simulink model "rtwdemo_basicsc"  (Simulink 7.6)
settings: Solver=FixedStepDiscrete  StartTime=0.0  StopTime=10.0  FixedStep=1  RelTol=1e-3
PostLoadFcn:
  | open_system('rtwdemo_basicsc/Auto');
values from neighbouring files (symbols this model uses):
  K1 = 3    [rtwdemo_cgv_init.m]    (also in rtwdemo_dow_data.m)
undefined symbols (not defined in the file or in its folder): LOWER, T1Break, T1Data, T2Data, UPPER
libraries: rtwdemowidgets x2
Description:
  | Specifying Storage Class Within a Diagram
settings Model: Creator=The MathWorks Inc.  CovMetricSettings=d  ExtModeAutoUpdateStatusClock=off
settings MATStruct: SampleTime=1  Offset=0  Priority=[20.0]
settings DataIOCC: SignalLoggingName=sigsOut
settings OptimizationCC: InlineParams=on  InlineInvariantSignals=on  StateBitsets=on  DataBitsets=on  UseTempVars=on  EfficientFloat2IntCast=on  EfficientMapNaN2IntZero=off
settings DebuggingCC: CheckExecutionContextPreStartOutputMsg=on  CheckExecutionContextRuntimeOutputMsg=on  SolverPrmCheckMsg=none  ParameterUnderflowMsg=error  ParameterPrecisionLossMsg=none  StrictBusMsg=ErrorOnBusTreatedAsVector
settings HardwareCC: ProdIntDivRoundTo=Zero  ProdEndianess=LittleEndian  ProdHWDeviceType=Generic->32-bit Embedded Processor  TargetHWDeviceType=Generic->32-bit Embedded Processor
settings SFSimCC: SimParseCustomCode=off
settings RTWCC: TLCOptions=-p0  GenerateReport=on  RTWVerbose=off  ProcessScript=grt_make_rtw_hook  LaunchReport=on
settings GRTTargetCC: TargetFcnLib=ansi_tfl_tmw.mat

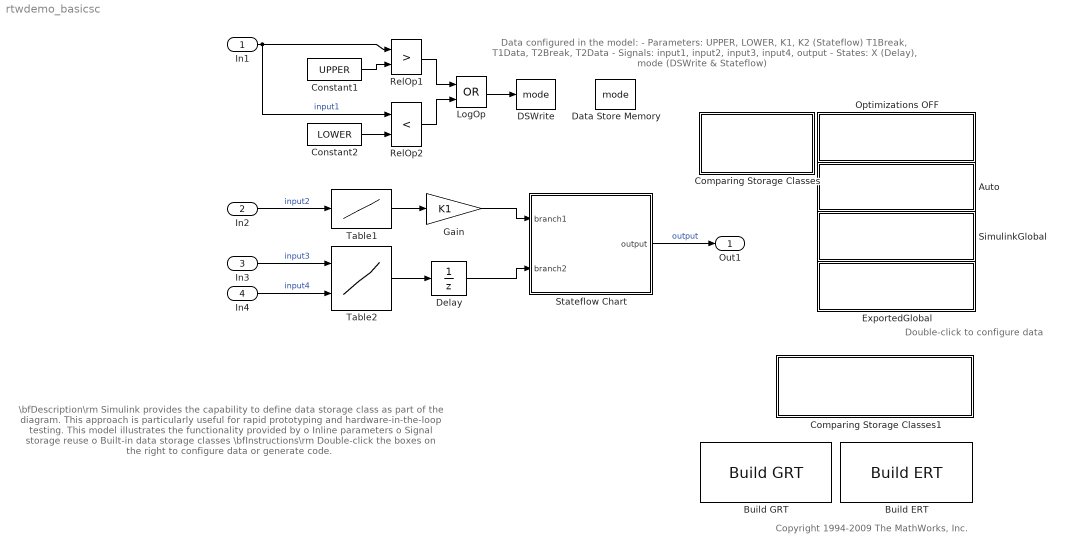
== system rtwdemo_basicsc ==
  note: Data configured in the model:
      | - Parameters: UPPER, LOWER, K1, K2 (Stateflow)
      |   T1Break, T1Data, T2Break, T2Data
      | - Signals: input1, input2, input3, input4, output
      | - States: X (Delay), mode (DSWrite & Stateflow)
  note: Double-click to configure data
  note: \bfDescription\rm
      | Simulink provides the capability to define data storage class as part of
      | the diagram. This approach is particularly useful for rapid prototyping
      | and hardware-in-the-loop testing.
      |
      | This model illustrates the functionality provided by
      | o Inline parameters
      | o Signal storage reuse
      | o Built-in data storage classes
      |
      | \bfInstructions\rm
      | Double-click the boxes on the right to configure data or generate code.
  note: Copyright 1994-2009 The MathWorks, Inc.
  In1 : Inport  OutDataTypeStr=single  PortDimensions=1  SampleTime=1
  In2 : Inport  Port=2  OutDataTypeStr=single  PortDimensions=1  SampleTime=1
  In3 : Inport  Port=3  OutDataTypeStr=single  PortDimensions=1  SampleTime=1
  In4 : Inport  Port=4  OutDataTypeStr=single  PortDimensions=1  SampleTime=1
  Auto : Subsystem  mask(Basic data packaging - configure model){Optimizations=on, StorageClass=Auto, DataInitFcn=rtwdemo_basicsc_config}
      mask prompts: Optimizations "Use Optimizations"
      mask help: OpenFcn configures model for data packaging demo.
      mask init:
      | if strcmp(Optimizations, 'on')
      |   dispStr = [StorageClass, '\nStorage Class'];
      | else
      |   set_param(gcb, 'StorageClass', 'Auto');
      |   dispStr = ['InlineParameters OFF\n', ...
      | 		     'SignalStorageReuse OFF'];
      | end
      settings: OpenFcn=feval(get_param(gcb, 'DataInitFcn'), bdroot(gcb), get_param(gcb, 'Optimizations'), get_param(gcb, 'StorageClass'));
      mask StyleString: checkbox,popup(Auto|SimulinkGlobal|ExportedGlobal),edit
      mask CallbackString:
      | if strcmp(get_param(gcb, 'Optimizations'), 'off')
      |   set_param(gcb, 'MaskEnableString', 'on,off,on');
      | else
      |   set_param(gcb, 'MaskEnableString', 'on,on,on');
      | end||
      mask Display: disp(dispStr);
  Build ERT : rtwdemowidgets/Build ERT  SystemSampleTime=-1  attrib_overrides={'InlineParams', 'OptimizeBlockIOStorage'}
  Build GRT : rtwdemowidgets/Build GRT  SystemSampleTime=-1  attrib_overrides={'InlineParams', 'OptimizeBlockIOStorage'}
  Comparing Storage Classes : Subsystem
      mask Display: disp(['Compare the\noptions ..', '.\n(double-click)']);
  Comparing Storage Classes1 : Subsystem
      settings: OpenFcn=rtwdemo_advsc
      mask Display: disp(['Advanced data packaging using\nSimulink data objects ..', '.\n(double-click)']);
  Constant1 : Constant  Value=UPPER  OutDataTypeStr=Inherit: Inherit via back propagation
  Constant2 : Constant  Value=LOWER  OutDataTypeStr=Inherit: Inherit via back propagation
  DSWrite : DataStoreWrite  DataStoreName=mode
  Data Store Memory : DataStoreMemory  DataStoreName=mode  OutDataTypeStr=boolean
  Delay : UnitDelay  StateIdentifier=X
  ExportedGlobal : Subsystem  mask(Basic data packaging - configure model){Optimizations=on, StorageClass=ExportedGlobal, DataInitFcn=rtwdemo_basicsc_config}
      mask prompts: Optimizations "Use Optimizations"
      mask help: OpenFcn configures model for data packaging demo.
      mask init: same as rtwdemo_basicsc/Auto
      settings: OpenFcn=feval(get_param(gcb, 'DataInitFcn'), bdroot(gcb), get_param(gcb, 'Optimizations'), get_param(gcb, 'StorageClass'));
      mask StyleString: checkbox,popup(Auto|SimulinkGlobal|ExportedGlobal),edit
      mask CallbackString:
      | if strcmp(get_param(gcb, 'Optimizations'), 'off')
      |   set_param(gcb, 'MaskEnableString', 'on,off,on');
      | else
      |   set_param(gcb, 'MaskEnableString', 'on,on,on');
      | end||
      mask Display: disp(dispStr);
  Gain : Gain  Gain=K1  SaturateOnIntegerOverflow=on  OutDataTypeStr=Inherit: Same as input  ParamDataTypeStr=Inherit: Same as input
  LogOp : Logic  Operator=OR
  Optimizations OFF : Subsystem  mask(Basic data packaging - configure model){Optimizations=off, StorageClass=Auto, DataInitFcn=rtwdemo_basicsc_config}
      mask prompts: Optimizations "Use Optimizations"
      mask help: OpenFcn configures model for data packaging demo.
      mask init: same as rtwdemo_basicsc/Auto
      settings: OpenFcn=feval(get_param(gcb, 'DataInitFcn'), bdroot(gcb), get_param(gcb, 'Optimizations'), get_param(gcb, 'StorageClass'));
      mask StyleString: checkbox,popup(Auto|SimulinkGlobal|ExportedGlobal),edit
      mask CallbackString:
      | if strcmp(get_param(gcb, 'Optimizations'), 'off')
      |   set_param(gcb, 'MaskEnableString', 'on,off,on');
      | else
      |   set_param(gcb, 'MaskEnableString', 'on,on,on');
      | end||
      mask Display: disp(dispStr);
  RelOp1 : RelationalOperator  Operator=>  InputSameDT=on
  RelOp2 : RelationalOperator  Operator=<  InputSameDT=on
  SimulinkGlobal : Subsystem  mask(Basic data packaging - configure model){Optimizations=on, StorageClass=SimulinkGlobal, DataInitFcn=rtwdemo_basicsc_config}
      mask prompts: Optimizations "Use Optimizations"
      mask help: OpenFcn configures model for data packaging demo.
      mask init: same as rtwdemo_basicsc/Auto
      settings: OpenFcn=feval(get_param(gcb, 'DataInitFcn'), bdroot(gcb), get_param(gcb, 'Optimizations'), get_param(gcb, 'StorageClass'));
      mask StyleString: checkbox,popup(Auto|SimulinkGlobal|ExportedGlobal),edit
      mask CallbackString:
      | if strcmp(get_param(gcb, 'Optimizations'), 'off')
      |   set_param(gcb, 'MaskEnableString', 'on,off,on');
      | else
      |   set_param(gcb, 'MaskEnableString', 'on,on,on');
      | end||
      mask Display: disp(dispStr);
  Stateflow Chart : Stateflow chart  TreatAsAtomicUnit=on
  Table1 : Lookup  InputValues=T1Break  Table=T1Data  SaturateOnIntegerOverflow=on
  Table2 : Lookup2D  RowIndex=T2Break  ColumnIndex=T2Break  Table=T2Data  InputSameDT=on
  Out1 : Outport
  wires:
  RelOp1/1 -> LogOp/1
  RelOp2/1 -> LogOp/2
  Constant2/1 -> RelOp2/2
  In2/1 -> Table1/1  "input2"
  Gain/1 -> Stateflow Chart/1(branch1)
  Table1/1 -> Gain/1
  Table2/1 -> Delay/1
  Constant1/1 -> RelOp1/2
  In1/1 -> RelOp2/1, RelOp1/1  "input1"
  In3/1 -> Table2/1  "input3"
  In4/1 -> Table2/2  "input4"
  Stateflow Chart/1(output) -> Out1/1  "output"
  Delay/1 -> Stateflow Chart/2(branch2)
  LogOp/1 -> DSWrite/1

== system rtwdemo_basicsc/Auto ==

== system rtwdemo_basicsc/Comparing Storage Classes ==
  note: 4. Unstructured storage classes (e.g., ExportedGlobal):
      |
      | Motivation:
      | - Interface to global data in hand-written (legacy) code
      |
      | Behavior:
      | - Select parameters and signals are global, unstructured variables
      | - Select states and root-level I/O are global, unstructured variables
      |
      | Advantages:
      | - Data names are preserved in the generated code
      |
      | Disadvantages:
      | - Imposes certain modeling restrictions
      | - Disables certain code optimizations
  note: 3. SimulinkGlobal storage class:
      |
      | Motivation:
      | - Provide visibility (persistence) for selected data
      |
      | Behavior:
      | - Select parameters and signals are members of persistent data structures
      | - All states and root-level I/O are members of persistent data structures
      |
      | Advantages:
      | - Only increase memory usage for data of interest
      | - Provides visibility to data without limitations
      |
      | Disadvantages:
      | - Minimal control over variable names
      |
      | How to specify SimulinkGlobal:
      | - Parameters: Tunable + Auto storage class
      | - Signals: Test point + Auto storage class
      | - States: Auto storage class
  note: 2. Auto storage class:
      |
      | Motivation:
      | - Maximize efficiency of the generated code
      |
      | Behavior:
      | - Parameters are inlined and intermediate signals are eliminated
      | - All states and root-level I/O are members of persistent data structures
      |
      | Advantages:
      | - Optimized code generation
      | - Default behavior when optimizations enabled (easy to use)
      |
      | Disadvantages:
      | - Parameters and signals do not appear as variables in the generated code
  note: 1. Inline parameters and signal storage reuse OFF:
      |
      | Motivation:
      | - Provide visibility (persistence) for all data
      | - Useful for simulation and rapid prototyping
      |
      | Behavior:
      | - All parameters and signals are members of persistent data structures
      | - All states and root-level I/O are members of persistent data structures
      |
      | Advantages:
      | - Easy access to data via model-wide settings
      |
      | Disadvantages:
      | - Generated code is non-optimal
      | - Minimal control over variable names
  note: NOTE: Descriptions 2-4 assume that the inline parameters and signal storage reuse optimizations are ON.

== system rtwdemo_basicsc/Comparing Storage Classes1 ==

== system rtwdemo_basicsc/ExportedGlobal ==

== system rtwdemo_basicsc/Optimizations OFF ==

== system rtwdemo_basicsc/SimulinkGlobal ==

== stateflow chart Stateflow Chart ==
  note: This chart implements an if-else condition, based
      | on the value of data store memory "mode".
      | The result is multiplied by parameter "K2".
      |
      | Using a Simulink switch (or if-action) and gain block,
      |     results in virtually identical code.
  (junction 7) -> (junction 4) : {output = branch1;}
  (junction 4) -> (junction 6) : {output *= K2;}
  (junction 5) -> (junction 4) [order 2] : {output = branch2;}
  (default) -> (junction 5)
  (junction 5) -> (junction 7) [order 1] : [mode]
  data: branch1 input double; mode data_store_memory double; branch2 input double; output output type(branch1) size=size(branch1); K2 parameter double
